simulink model "power_hvdc12pulse"  (Simulink 6.0)
settings: Solver=FixedStepDiscrete  SolverMode=SingleTasking  StartTime=0.0  StopTime=2  FixedStep=Ts  RelTol=1e-3  AbsTol=1e-2
InitFcn:
  | Ts=50e-6;
undefined symbols (not defined in the file or in its folder): CLARK, Current, D1, Delta, DiscIntNeverNeededParam, Gamma, Inverter, lag, lib_mesures, Voltage, Yg
libraries: powerlib x39, powerlib_extras x30, simulink x3
(part 1 of 3)
Description:
  | The 'Model  initialization function' defined in the
  | 
  | Model Properties automatically sets the sample time
  | 
  | Ts to 50e-6 s
settings Model: Creator=Gilbert Sybille, IREQ  LastModifiedBy=batserve  ExtModeTrigMode=oneshot  ExtModeArmWhenConnect=off  ExtModeAutoUpdateStatusClock=off
settings DataIOCC: LimitDataPoints=off  SaveTime=off  SignalLoggingName=sigsOut
settings OptimizationCC: BlockReduction=off  BooleanDataType=off
settings DebuggingCC: CheckExecutionContextPreStartOutputMsg=on  CheckExecutionContextRuntimeOutputMsg=on  SolverPrmCheckMsg=none  UnconnectedInputMsg=none  UnconnectedOutputMsg=none
settings HardwareCC: TargetUnknown=on

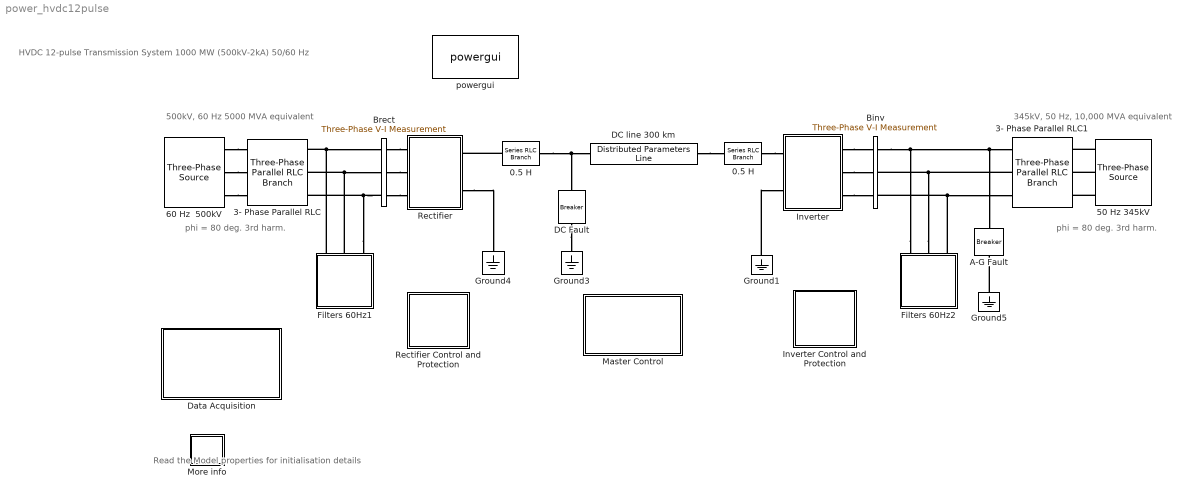
== system power_hvdc12pulse ==
  note: phi = 80 deg. 3rd harm.
  note: HVDC 12-pulse Transmission System
      | 1000 MW (500kV-2kA)   50/60 Hz
  note: 500kV, 60 Hz
      |  5000 MVA equivalent
  note: 345kV, 50 Hz,
      | 10,000 MVA equivalent
  note: phi = 80 deg. 3rd harm.
  note: Read the Model properties
      | for initialisation details
  " 50 Hz 345kV  " : powerlib/Electrical Sources/Three-Phase Source  Orientation=left  Voltage=345e3  PhaseAngle=0  Frequency=50  InternalConnection=Yg  SpecifyImpedance=off  Resistance=0  Inductance=28.0e-3  ShortCircuitLevel=0  BaseVoltage=0  XRratio=0
  " 60 Hz  500kV" : powerlib/Electrical Sources/Three-Phase Source  Voltage=500e3  PhaseAngle=0  Frequency=60  InternalConnection=Yg  SpecifyImpedance=off  Resistance=0  Inductance=98.03e-3  ShortCircuitLevel=0  BaseVoltage=0  XRratio=0
  0.5 H : powerlib/Elements/Series RLC Branch  PhysicalDomain=powersysdomain  SubClassName=unknown  LeftPortType=p1  RightPortType=p1  LConnTagsString=__new0  RConnTagsString=__new0  Resistance=1  Inductance=0.5  Capacitance=inf  Measurements=None
  "0.5 H " : powerlib/Elements/Series RLC Branch  Orientation=left  PhysicalDomain=powersysdomain  SubClassName=unknown  LeftPortType=p1  RightPortType=p1  LConnTagsString=__new0  RConnTagsString=__new0  Resistance=1  Inductance=0.5  Capacitance=inf  Measurements=None
  3- Phase Parallel RLC : powerlib/Elements/Three-Phase Parallel RLC Branch  PhysicalDomain=powersysdomain  SubClassName=unknown  LeftPortType=p1  RightPortType=p1  LConnTagsString=A|B|C  RConnTagsString=A|B|C  Resistance=26.07  Inductance=48.86e-3  Capacitance=0  Measurements=None
  3- Phase Parallel RLC1 : powerlib/Elements/Three-Phase Parallel RLC Branch  Orientation=left  PhysicalDomain=powersysdomain  SubClassName=unknown  LeftPortType=p1  RightPortType=p1  LConnTagsString=A|B|C  RConnTagsString=A|B|C  Resistance=6.205  Inductance=13.96e-3  Capacitance=0  Measurements=None
  A-G Fault : powerlib/Elements/Breaker  Orientation=down  BreakerResistance=0.01  InitialState=0  SnubberResistance=inf  SnubberCapacitance=inf  SwitchingTimes=[ 0.7 0.8]*100  External=off  Measurements=Branch current
      settings: AttributesFormatString=\n
  Binv : powerlib/Measurements/Three-Phase V-I Measurement  Orientation=left  VoltageMeasurement=phase-to-ground  SetLabelV=on  LabelV=Vabc_I  Vpu=on  Vbase=345e3  CurrentMeasurement=yes  SetLabelI=on  LabelI=Iabc_I  Ipu=on  Pbase=100e6  OutputType=Magnitude  PhasorSimulation=off  PSBequivalent=0
  Brect : powerlib/Measurements/Three-Phase V-I Measurement  VoltageMeasurement=phase-to-ground  SetLabelV=on  LabelV=Vabc_R  Vpu=on  Vbase=500e3  CurrentMeasurement=yes  SetLabelI=on  LabelI=Iabc_R  Ipu=on  Pbase=100e6  OutputType=Magnitude  PhasorSimulation=off  PSBequivalent=0
  DC Fault : powerlib/Elements/Breaker  Orientation=down  BreakerResistance=1  InitialState=0  SnubberResistance=inf  SnubberCapacitance=inf  SwitchingTimes=[0.7 0.75]*100  External=off  Measurements=Branch current
      settings: AttributesFormatString=\n
  DC line 300 km : powerlib/Elements/Distributed Parameters Line  Phases=1  Frequency=60  Resistance=0.015  Inductance=0.792e-3  Capacitance=14.4e-9  Length=300  x1=[0 -2.16105063708639e-012;0.000202625960824372 -2.78820694913162e-012;0.000405251921648744 -3.41415596345104e-012;0.000607877882473116 -4.03596541237589e-012;0.000810503843297489 -4.65066327836032e-012;0.00101312980412186 -5.25525247617399e-012]  x2=[0 -1.28636510443273e-012;0.000202625960824372 -1.90237836086429e-012;0.000405251921648744 -2.52160651295295e-012;0.000607877882473116 -3.14111601303326e-012;0.000810503843297489 -3.75791095814674e-012;0.00101312980412186 -4.36894806263535e-012]  x3=[0 -5.39692178751901e-015;0.000202625960824372 -7.25920757796091e-015;0.000405251921648744 -9.14272797774125e-015;0.000607877882473116 -1.10394956670709e-014;0.000810503843297489 -1.29411763980793e-014;0.00101312980412186 -1.48391265509203e-014]  x4=[0 4.1267112956018e-015;0.000202625960824372 8.19507726484828e-016;0.000405251921648744 -2.53679729362182e-015;0.000607877882473116 -5.92679713170551e-015;0.000810503843297489 -9.33469221052342e-015;0.00101312980412186 -1.27443660669749e-014]  x5=0.00101312980412186  Measurements=Phase-to-ground voltages
      settings: AttributesFormatString=\n
  Data Acquisition : Subsystem
      mask Display: disp('Open this block\nto visualize\nrecorded signals')
  Filters 60Hz1 : Subsystem  Orientation=down
      mask Display: disp('AC filters \n60 Hz\n600 Mvar')
  Filters 60Hz2 : Subsystem  Orientation=down
      mask Display: disp('AC filters \n50 Hz\n600 Mvar')
  Ground{1,3..5} (4 alike) : powerlib/Elements/Ground  Orientation=down  PhysicalDomain=powersysdomain  SubClassName=unknown  LeftPortType=p1  RightPortType=p1  LConnTagsString=a
  Inverter : Subsystem  Orientation=left
  Inverter Control and Protection : Subsystem  Orientation=left
  Master Control : Subsystem
      mask Display: disp('Master Control')
  More info : Subsystem
      mask Display: disp('?')
  Rectifier : Subsystem
  Rectifier Control and Protection : Subsystem
  powergui : powerlib/powergui  Priority=2  Frange=[0:2:500]  Ylog=off  Xlog=on  save=off  variable=ZData  ZoomFFT=on  StartTime=0.0  cycles=1  DisplayStyle=off  fundamental=60  FreqAxis=off  MaxFrequency=1000  frequencyindice=1  frequencyindicesteady=1  RmsSteady=1  display=off  Ts=Ts  methode=off  frequency=60  echomessages=on
  connections:
  DC Fault/RConn1 -- Ground3/LConn1
  " 60 Hz  500kV"/RConn1 -- 3- Phase Parallel RLC/LConn1
  " 60 Hz  500kV"/RConn2 -- 3- Phase Parallel RLC/LConn2
  " 60 Hz  500kV"/RConn3 -- 3- Phase Parallel RLC/LConn3
  Filters 60Hz1/LConn2 -- 3- Phase Parallel RLC/RConn2 -- Brect/LConn2
  Filters 60Hz1/LConn3 -- Brect/LConn3 -- 3- Phase Parallel RLC/RConn3
  " 50 Hz 345kV  "/RConn2 -- 3- Phase Parallel RLC1/LConn2
  " 50 Hz 345kV  "/RConn1 -- 3- Phase Parallel RLC1/LConn1
  " 50 Hz 345kV  "/RConn3 -- 3- Phase Parallel RLC1/LConn3
  Filters 60Hz2/LConn1 -- 3- Phase Parallel RLC1/RConn1 -- A-G Fault/LConn1 -- Binv/LConn1
  Filters 60Hz2/LConn2 -- 3- Phase Parallel RLC1/RConn2 -- Binv/LConn2
  Filters 60Hz2/LConn3 -- 3- Phase Parallel RLC1/RConn3 -- Binv/LConn3
  Filters 60Hz1/LConn1 -- 3- Phase Parallel RLC/RConn1 -- Brect/LConn1
  Rectifier/RConn2 -- Ground4/LConn1
  Ground1/LConn1 -- Inverter/RConn2
  Ground5/LConn1 -- A-G Fault/RConn1
  Inverter/LConn1 -- Binv/RConn1
  Inverter/LConn2 -- Binv/RConn2
  Inverter/LConn3 -- Binv/RConn3
  Brect/RConn1 -- Rectifier/LConn1
  Brect/RConn2 -- Rectifier/LConn2
  Brect/RConn3 -- Rectifier/LConn3
  0.5 H/LConn1 -- Rectifier/RConn1
  DC line 300 km/RConn1 -- "0.5 H "/RConn1
  "0.5 H "/LConn1 -- Inverter/RConn1
  0.5 H/RConn1 -- DC line 300 km/LConn1 -- DC Fault/LConn1

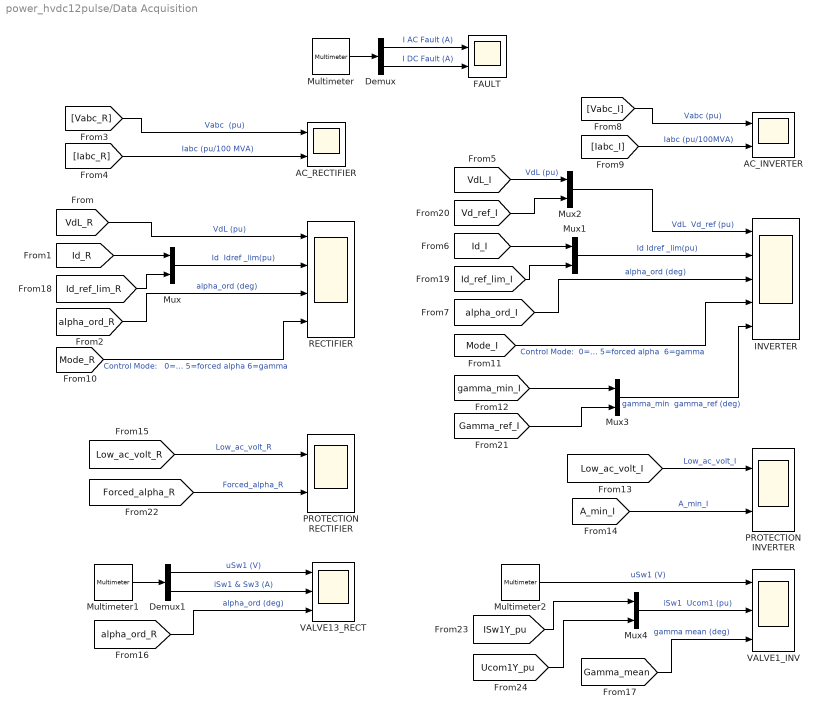
== system power_hvdc12pulse/Data Acquisition ==
  AC_INVERTER : Scope  NumInputPorts=2
      settings: YMin=-1.25~-50  YMax=1.5~20  SaveName=VI_abc_inv  Decimation=Ts  SampleInput=on  SampleTime=Ts
  AC_RECTIFIER : Scope  NumInputPorts=2
      settings: TimeRange=0.2008622476996453  YMin=-1~-25  YMax=1~30  DataFormat=Array  Decimation=Ts  SampleInput=on  SampleTime=Ts
  Demux : Demux  Outputs=2
  Demux1 : Demux  Outputs=[1 2]
  FAULT : Scope  NumInputPorts=2
      settings: YMin=-1~-1000  YMax=1~8000  Decimation=Ts  SampleInput=on  SampleTime=Ts
  INVERTER : Scope  NumInputPorts=5
      settings: TimeRange=2  YMin=-0.5~-0.5~50~0~0  YMax=1.5~1.5~200~6~200  SaveName=inv  Decimation=Ts  SampleInput=on  SampleTime=Ts
  Multimeter : powerlib/Measurements/Multimeter  Tag=PoWeRsYsTeMmEaSuReMeNt  PhasorSimulation=off  OutputType=Magnitude  sel=[23 24]  L=42  Gain=[1 1]  yselected={'Ib: A-G Fault','Ib: DC Fault'};  PSBOutputType=1  PSBequivalent=0  AxesSetting=[0,0.1,-100,100]  Display=0  SavedBlockNames={}
      settings: AttributesFormatString=\n
  Multimeter1 : powerlib/Measurements/Multimeter  Tag=PoWeRsYsTeMmEaSuReMeNt  PhasorSimulation=off  OutputType=Magnitude  sel=[11 37 39]  L=42  Gain=[1 1 1]  yselected={'Usw1: Rectifier/Rectifier/Bridge Y','Isw1: Rectifier/Rectifier/Bridge Y','Isw3: Rectifier/Rectifier/Bridge Y'};  PSBOutputType=1  PSBequivalent=0  AxesSetting=[0,0.1,-100,100]  Display=0  SavedBlockNames={}
      settings: AttributesFormatString=\n
  Multimeter2 : powerlib/Measurements/Multimeter  Tag=PoWeRsYsTeMmEaSuReMeNt  PhasorSimulation=off  OutputType=Magnitude  sel=1  L=42  Gain=1  yselected={'Usw1: Inverter/Inverter/Bridge Y'};  PSBOutputType=1  PSBequivalent=0  AxesSetting=[0,0.1,-100,100]  Display=0  SavedBlockNames={}
      settings: AttributesFormatString=\n
  Mux{,1..4} (5 alike) : Mux  Inputs=2
  PROTECTION INVERTER : Scope  NumInputPorts=2
      settings: YMin=-1~2.71051e-020  YMax=1~0.0007  SaveName=ScopeData2  DataFormat=Array  Decimation=Ts  SampleInput=on  SampleTime=Ts
  PROTECTION RECTIFIER : Scope  NumInputPorts=2
      settings: YMin=-1.25~-5  YMax=1.25~5  SaveName=ScopeData5  DataFormat=Array  Decimation=Ts  SampleInput=on  SampleTime=Ts
  RECTIFIER : Scope  NumInputPorts=4
      settings: YMin=-0.5~-0.1~0~0  YMax=1.25~1.1~175~5  SaveName=rect  Decimation=Ts  SampleInput=on  SampleTime=Ts
  VALVE13_RECT : Scope  NumInputPorts=3
      settings: YMin=-400000~-500~10  YMax=400000~2500~100  SaveName=ScopeData3  Decimation=Ts  SampleInput=on  SampleTime=Ts
  VALVE1_INV : Scope  NumInputPorts=3
      settings: YMin=-200000~-2~-1  YMax=350000~2~1  SaveName=ScopeData6  Decimation=Ts  SampleInput=on  SampleTime=Ts
  wires:
  [Mode_R] -> RECTIFIER/4  "Control Mode:   0=blocked  1=current 2=voltage 3=alpha min  4=alpha max 5=forced alpha 6=gamma"
  Demux/2 -> FAULT/2  "I DC Fault (A)"
  Demux/1 -> FAULT/1  "I AC Fault (A)"
  [alpha_ord_I] -> INVERTER/3  "alpha_ord (deg)"
  [Iabc_I] -> AC_INVERTER/2  "Iabc (pu/100MVA)"
  [Vabc_I] -> AC_INVERTER/1  "Vabc (pu)"
  [alpha_ord_R] -> RECTIFIER/3  "alpha_ord (deg)"
  [VdL_R] -> RECTIFIER/1  "VdL (pu)"
  [Iabc_R] -> AC_RECTIFIER/2  "Iabc (pu/100 MVA)"
  [Vabc_R] -> AC_RECTIFIER/1  "Vabc  (pu)"
  Multimeter/1 -> Demux/1
  [Low_ac_volt_I] -> PROTECTION INVERTER/1  "Low_ac_volt_I"
  [A_min_I] -> PROTECTION INVERTER/2  "A_min_I"
  [Low_ac_volt_R] -> PROTECTION RECTIFIER/1  "Low_ac_volt_R"
  Mux/1 -> RECTIFIER/2  "Id  Idref _lim(pu)"
  [Id_R] -> Mux/1
  [Id_ref_lim_R] -> Mux/2
  [Id_I] -> Mux1/1
  [Id_ref_lim_I] -> Mux1/2
  Mux1/1 -> INVERTER/2  "Id Idref _lim(pu)"
  [Mode_I] -> INVERTER/4  "Control Mode:  0=blocked  1=current  2=voltage  3=alpha min  4=alpha max  5=forced alpha  6=gamma"
  [VdL_I] -> Mux2/1  "VdL (pu)"
  Mux2/1 -> INVERTER/1  "VdL  Vd_ref (pu)"
  [Vd_ref_I] -> Mux2/2
  [gamma_min_I] -> Mux3/1
  Mux3/1 -> INVERTER/5  "gamma_min  gamma_ref (deg)"
  [Gamma_ref_I] -> Mux3/2
  [Forced_alpha_R] -> PROTECTION RECTIFIER/2  "Forced_alpha_R"
  Multimeter1/1 -> Demux1/1
  Demux1/1 -> VALVE13_RECT/1  "uSw1 (V)"
  Demux1/2 -> VALVE13_RECT/2  "iSw1 & Sw3 (A)"
  [alpha_ord_R] -> VALVE13_RECT/3  "alpha_ord (deg)"
  Multimeter2/1 -> VALVE1_INV/1  "uSw1 (V)"
  [Gamma_mean] -> VALVE1_INV/3  "gamma mean (deg)"
  Mux4/1 -> VALVE1_INV/2  "iSw1  Ucom1 (pu)"
  [ISw1Y_pu] -> Mux4/1
  [Ucom1Y_pu] -> Mux4/2

== system power_hvdc12pulse/Filters 60Hz1 ==
  note: Capacitor banks
  note: Tuned filters
  note: High-pass
      | damped filter
  note: 60 Hz filters 4*150 Mvars @ 500 kV
  11th 150 Mvar Q=100 : powerlib/Elements/Three-Phase Harmonic Filter  Orientation=down  PhysicalDomain=powersysdomain  SubClassName=unknown  LeftPortType=p1  RightPortType=p1  LConnTagsString=A|B|C  FilterType=Single-tuned  FilterConnection=Y (grounded)  ParNom=[500e3 60]  Qc=150e6  Fr=[11*60]  Frd=[11*60 13*60]  Q=100  Measurements=None
      settings: AttributesFormatString=\n
  "13th 150 Mvar Q=100 " : powerlib/Elements/Three-Phase Harmonic Filter  Orientation=down  PhysicalDomain=powersysdomain  SubClassName=unknown  LeftPortType=p1  RightPortType=p1  LConnTagsString=A|B|C  FilterType=Single-tuned  FilterConnection=Y (grounded)  ParNom=[500e3 60]  Qc=150e6  Fr=[13*60]  Frd=[11*60 13*60]  Q=100  Measurements=None
      settings: AttributesFormatString=\n
  150 Mvar : powerlib/Elements/Three-Phase Series RLC Load  Orientation=down  PhysicalDomain=powersysdomain  SubClassName=unknown  LeftPortType=p1  RightPortType=p1  LConnTagsString=A|B|C  Configuration=Y (grounded)  NominalVoltage=500e3  NominalFrequency=60  ActivePower=0  InductivePower=0  CapacitivePower=150e6  Measurements=None
  24th 150 Mvar Q=3 : powerlib/Elements/Three-Phase Harmonic Filter  Orientation=down  PhysicalDomain=powersysdomain  SubClassName=unknown  LeftPortType=p1  RightPortType=p1  LConnTagsString=A|B|C  FilterType=High-pass  FilterConnection=Y (grounded)  ParNom=[500e3 60]  Qc=150e6  Fr=[24*60]  Frd=[11*60 13*60]  Q=3  Measurements=None
      settings: AttributesFormatString=\n
  A : PMIOPort  Orientation=down  Port=1  Side=Left
  B : PMIOPort  Orientation=down  Port=2  Side=Left
  C : PMIOPort  Orientation=down  Port=3  Side=Left
  connections:
  150 Mvar/LConn3 -- 24th 150 Mvar Q=3/LConn3 -- "13th 150 Mvar Q=100 "/LConn3 -- 11th 150 Mvar Q=100/LConn3 -- C/RConn1
  150 Mvar/LConn2 -- 24th 150 Mvar Q=3/LConn2 -- "13th 150 Mvar Q=100 "/LConn2 -- 11th 150 Mvar Q=100/LConn2 -- B/RConn1
  150 Mvar/LConn1 -- 24th 150 Mvar Q=3/LConn1 -- "13th 150 Mvar Q=100 "/LConn1 -- 11th 150 Mvar Q=100/LConn1 -- A/RConn1

== system power_hvdc12pulse/Filters 60Hz2 ==
  note: 50 Hz filters 4*150 Mvars @ 345 kV
  note: Tuned filters
  note: Capacitor banks
  note: High-pass
      | damped filter
  11th 150 Mvar Q=100 : powerlib/Elements/Three-Phase Harmonic Filter  Orientation=down  PhysicalDomain=powersysdomain  SubClassName=unknown  LeftPortType=p1  RightPortType=p1  LConnTagsString=A|B|C  FilterType=Single-tuned  FilterConnection=Y (grounded)  ParNom=[345e3 50]  Qc=150e6  Fr=[11*50]  Frd=[11*60 13*60]  Q=100  Measurements=None
      settings: AttributesFormatString=\n
  "13th 150 Mvar Q=100 " : powerlib/Elements/Three-Phase Harmonic Filter  Orientation=down  PhysicalDomain=powersysdomain  SubClassName=unknown  LeftPortType=p1  RightPortType=p1  LConnTagsString=A|B|C  FilterType=Single-tuned  FilterConnection=Y (grounded)  ParNom=[345e3 50]  Qc=150e6  Fr=[13*50]  Frd=[11*60 13*60]  Q=100  Measurements=None
      settings: AttributesFormatString=\n
  150 Mvar : powerlib/Elements/Three-Phase Series RLC Load  Orientation=down  PhysicalDomain=powersysdomain  SubClassName=unknown  LeftPortType=p1  RightPortType=p1  LConnTagsString=A|B|C  Configuration=Y (grounded)  NominalVoltage=345e3  NominalFrequency=50  ActivePower=0  InductivePower=0  CapacitivePower=150e6  Measurements=None
  24th 150 Mvar Q=3 : powerlib/Elements/Three-Phase Harmonic Filter  Orientation=down  PhysicalDomain=powersysdomain  SubClassName=unknown  LeftPortType=p1  RightPortType=p1  LConnTagsString=A|B|C  FilterType=High-pass  FilterConnection=Y (grounded)  ParNom=[345e3 50]  Qc=150e6  Fr=[24*50]  Frd=[11*60 13*60]  Q=3  Measurements=None
      settings: AttributesFormatString=\n
  A : PMIOPort  Orientation=down  Port=1  Side=Left
  B : PMIOPort  Orientation=down  Port=2  Side=Left
  C : PMIOPort  Orientation=down  Port=3  Side=Left
  connections:
  150 Mvar/LConn1 -- 24th 150 Mvar Q=3/LConn1 -- "13th 150 Mvar Q=100 "/LConn1 -- 11th 150 Mvar Q=100/LConn1 -- A/RConn1
  150 Mvar/LConn2 -- 24th 150 Mvar Q=3/LConn2 -- "13th 150 Mvar Q=100 "/LConn2 -- 11th 150 Mvar Q=100/LConn2 -- B/RConn1
  150 Mvar/LConn3 -- 24th 150 Mvar Q=3/LConn3 -- "13th 150 Mvar Q=100 "/LConn3 -- 11th 150 Mvar Q=100/LConn3 -- C/RConn1

== system power_hvdc12pulse/Inverter ==
  1200 MVA : powerlib/Elements/Three-Phase Transformer (Three Windings)  Orientation=left  NominalPower=[ 1200e6 , 50 ]  Winding1Connection=Yg  Winding1="[ 345e3*0.96 0.0025  0 ]"  Winding2Connection=Y  Winding2="[ 200e3  0.0025 0.24]"  Winding3Connection=Delta (D1)  Winding3=[ 200e3 0.0025 0.24 ]  SetSaturation=off  Rm=500  Lm=500  Saturation="[0 0; 0.0024 1.2; 1.0  1.45]"  Hysteresis=off  DataFile='hysteresis'  SetInitialFlux=off  InitialFluxes=[-1.10749033878531 0.564800371868647 0.542689966916658]  Measurements=None  TransfoNumber=0
      settings: AttributesFormatString=\n
  A->pu : Gain  Orientation=left  Gain=1/2000  SaturateOnIntegerOverflow=on
  Id : powerlib/Measurements/Current Measurement  Tag=PoWeRsYsTeMmEaSuReMeNt  PhasorSimulation=off  OutputType=Magnitude  PSBequivalent=0
  Inverter : Subsystem  Orientation=left
      mask Display: plot(0,0,100,100,[30 70 50 30 ], [60 60 40 60], [50 50], [25 40], [50 50], [ 60 75], [30 70], [40 40], [50 60 70], [40 30 30]);
  A : PMIOPort  Orientation=left  Port=1  Side=Left
  B : PMIOPort  Orientation=left  Port=2  Side=Left
  C : PMIOPort  Orientation=left  Port=3  Side=Left
  + : PMIOPort  Port=4  Side=Right
  - : PMIOPort  Port=5  Side=Right
  tag scope: Id_I=global
  wires:
  [PulsesY_I] -> Inverter/1(Py)
  [PulsesD_I] -> Inverter/2(Pd)
  Id/1 -> A->pu/1
  A->pu/1 -> [Id_I]
  connections:
  C/RConn1 -- 1200 MVA/LConn3
  A/RConn1 -- 1200 MVA/LConn1
  -/RConn1 -- Inverter/RConn2
  Inverter/LConn6 -- 1200 MVA/RConn6
  1200 MVA/RConn5 -- Inverter/LConn5
  Inverter/LConn4 -- 1200 MVA/RConn4
  1200 MVA/RConn3 -- Inverter/LConn3
  Inverter/LConn2 -- 1200 MVA/RConn2
  1200 MVA/RConn1 -- Inverter/LConn1
  1200 MVA/LConn2 -- B/RConn1
  +/RConn1 -- Id/LConn1
  Id/RConn1 -- Inverter/RConn1

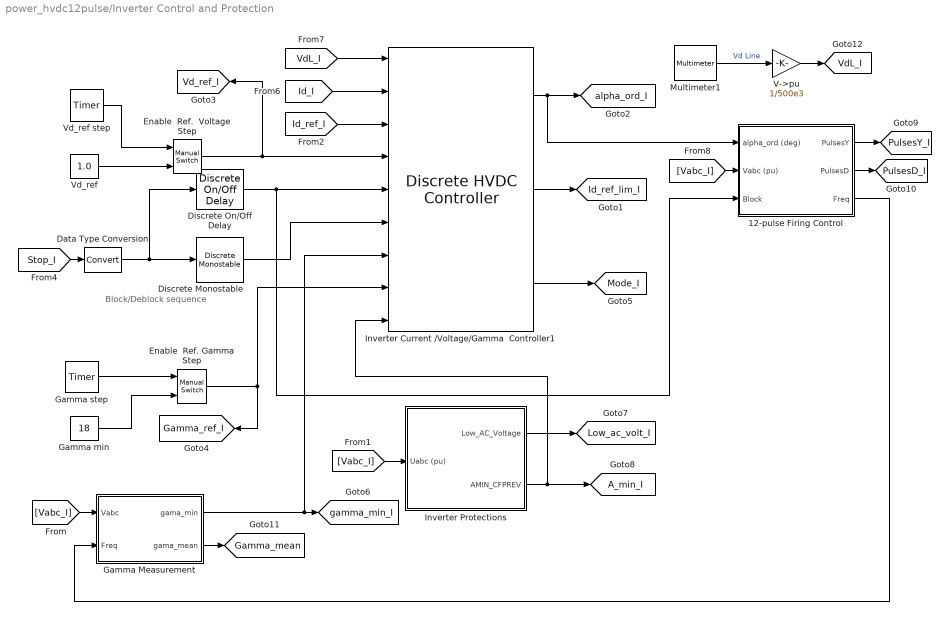
== system power_hvdc12pulse/Inverter Control and Protection ==
  note: Block/Deblock sequence
  12-pulse Firing Control : Subsystem  mask(HVDC Discrete 12-pulse Firing Control){Pw=101.5, PLL_PF=[0,  50], PLL_G=[60, 1400], dt=Ts}
      mask prompts: Pw "{Pulse Generator}: Pulse Width (deg)"; PLL_PF "{PLL}: Initial [Phase (deg) Frequency (Hz)]"; PLL_G "{PLL}: Regulator gains [Kp (rad)  Ki (rad/s)]"; dt "Sample Time (s):"
      mask help:
      | This block contains a PLL and a 12-pulse generator to provide the firing pulses to the HVDC converter.
      | The firing control is of the equidistant type. It is based on a Phase Locked Loop (PLL) synchronized on positive-sequence of the fundamental voltage.
      mask init:
      | PLL_ph = PLL_PF(1); PLL_f0 = PLL_PF(2);
      | PLL_Kp = PLL_G(1); PLL_Ki = PLL_G(2);
      mask Help:
      | INPUTS:
      | alpha :  Desired firing angle of thyristors (deg).
      | Vabc  : 3 phase-to-ground voltages (pu)  on the primary winding of the YgYD converter transformer
      | Block  : Logical signal  (0-1). The pulses are not generated when the value is 1.
      | 
      | 
      | 
      | OUTPUTS:
      |  PulsesY :  6 pulses to be sent to the half converter connected to the Wye winding.
      |  PulsesD :  6 pulses to be sent to the half converter connected to the Delta winding.
  Data Type Conversion : DataTypeConversion  OutDataTypeMode=boolean  SaturateOnIntegerOverflow=on  RndMeth=Zero
  Discrete Monostable : powerlib_extras/Discrete  Control Blocks/Discrete Monostable  EdgeDetect=Rising  t_mono=0.15  ic=1  Ts=Ts
  Discrete On/Off Delay : powerlib_extras/Discrete  Control Blocks/Discrete On//Off Delay  type_delay=On delay  delay=0.1  ic=1  Ts=Ts
  Enable  Ref.  Voltage Step : simulink/Signal Routing/Manual Switch  sw=1  action=0
  Enable  Ref. Gamma Step : simulink/Signal Routing/Manual Switch  sw=0  action=0
  Gamma Measurement : Subsystem
  Gamma min : Constant  Value=18
  Gamma step : powerlib_extras/Control  Blocks/Timer  t="[ 0  0.7  0.9  ]"  e="[ 18   23   18  ]"
  Inverter Current /Voltage/Gamma  Controller1 : powerlib_extras/Discrete  Control Blocks/Discrete HVDC Controller  Mode=Inverter (Current + Voltage + Gamma)  XPILim=[166, 92]  XLin=[160, 120]  XKPI_I=[45, 4500, 90]  Id_marg=0.1  XKPI_V="[35, 2250,  90]"  Vd_marg=0.05  XKPI_G="[1, 20,  90 ]"  G_marg=1  T_I=0.3e-3  XT_V="[15,  0.707]"  Xvdcol=[0.6, 0.18, 0.30, 0.1, 0.080]  alpha_const=off  Xalpha_fix=[92, inf, -1000]  dt=Ts
  Inverter Protections : Subsystem  TreatAsAtomicUnit=on
      mask Type: Protection LACVD a Radisson (cyc = 1 ms)
  Multimeter1 : powerlib/Measurements/Multimeter  Tag=PoWeRsYsTeMmEaSuReMeNt  PhasorSimulation=off  OutputType=Magnitude  sel=22  L=42  Gain=1  yselected={'Ur_ph1_gnd: DC line 300 km'};  PSBOutputType=1  PSBequivalent=0  AxesSetting=[0,0.1,-100,100]  Display=0  SavedBlockNames=-11
      settings: AttributesFormatString=\n
  V->pu : Gain  Gain=1/500e3  SaturateOnIntegerOverflow=on
  Vd_ref : Constant  Value=1.0
  Vd_ref step : powerlib_extras/Control  Blocks/Timer  t="[ 0  1  1.1  ]"  e="[ 1   0.9   1  ]"
  tag scope: A_min_I=global, Gamma_mean=global, Gamma_ref_I=global, Id_ref_lim_I=global, Low_ac_volt_I=global, Mode_I=global, PulsesD_I=global, PulsesY_I=global, VdL_I=global, Vd_ref_I=global, alpha_ord_I=global, gamma_min_I=global
  wires:
  Data Type Conversion/1 -> Discrete On/Off Delay/1, Discrete Monostable/1
  [Stop_I] -> Data Type Conversion/1
  [Vabc_I] -> Inverter Protections/1(Uabc (pu))
  Inverter Protections/2(AMIN_CFPREV) -> [A_min_I], Inverter Current /Voltage/Gamma  Controller1/9
  Inverter Protections/1(Low_AC_Voltage) -> [Low_ac_volt_I]
  V->pu/1 -> [VdL_I]
  Multimeter1/1 -> V->pu/1  "Vd Line"
  Enable  Ref. Gamma Step/1 -> [Gamma_ref_I], Inverter Current /Voltage/Gamma  Controller1/8
  Gamma step/1 -> Enable  Ref. Gamma Step/1
  Gamma min/1 -> Enable  Ref. Gamma Step/2
  Gamma Measurement/1(gama_min) -> [gamma_min_I], Inverter Current /Voltage/Gamma  Controller1/7
  [Vabc_I] -> Gamma Measurement/1(Vabc)
  Gamma Measurement/2(gama_mean) -> [Gamma_mean]
  12-pulse Firing Control/1(PulsesY) -> [PulsesY_I]
  12-pulse Firing Control/2(PulsesD) -> [PulsesD_I]
  Inverter Current /Voltage/Gamma  Controller1/1 -> [alpha_ord_I], 12-pulse Firing Control/1(alpha_ord (deg))
  Inverter Current /Voltage/Gamma  Controller1/2 -> [Id_ref_lim_I]
  Inverter Current /Voltage/Gamma  Controller1/3 -> [Mode_I]
  [Vabc_I] -> 12-pulse Firing Control/2(Vabc (pu))
  [VdL_I] -> Inverter Current /Voltage/Gamma  Controller1/1
  [Id_I] -> Inverter Current /Voltage/Gamma  Controller1/2
  [Id_ref_I] -> Inverter Current /Voltage/Gamma  Controller1/3
  Discrete On/Off Delay/1 -> 12-pulse Firing Control/3(Block), Inverter Current /Voltage/Gamma  Controller1/5
  Enable  Ref.  Voltage Step/1 -> Inverter Current /Voltage/Gamma  Controller1/4, [Vd_ref_I]
  Vd_ref/1 -> Enable  Ref.  Voltage Step/2
  Vd_ref step/1 -> Enable  Ref.  Voltage Step/1
  Discrete Monostable/1 -> Inverter Current /Voltage/Gamma  Controller1/6
  12-pulse Firing Control/3(Freq) -> Gamma Measurement/2(Freq)

== system power_hvdc12pulse/Master Control ==
  note: Master Control
  note: Balanced reference currents
  Constant : Constant  Value=0
  Enable  Ref. Current Step : simulink/Signal Routing/Manual Switch  sw=1  action=0
  Id_ref step : powerlib_extras/Control  Blocks/Timer  t="[ 0  0.7  0.8  ]"  e="[ 0   -0.2   0  ]"
  Informations : Subsystem
      mask Display: disp('?')
  Start/Stop : Subsystem  mask(Start/Stop  & Ramping  ){Min_ref=0.1, X_start=[0.3333, 0.02], X_up=[5.0, 0.4, 1.0], X_down=[-5.0,  1.4], T_stop=1.6}
      mask prompts: Min_ref "Minimum Steady-State Current Reference (pu):"; X_start "{Start Ramp}: [Rate (pu/s), Time (s)]"; X_up "{Up Ramp}: [Rate (pu/s), Time (s), Final Value (pu)]"; X_down "{Down Ramp}: [Rate (-pu/s), Time (s)]"; T_stop "Stop Time (s):"
      mask help:
      | At start-up, both converters are deblocked and ramped up to the minimum current (Minimum Steady-State Current Reference) with an adjustable rate (Start Ramp Rate) and application time (Start Ramp Time).
      |
      | After the system stabilisation the current is ramped up to its final value (Up Ramp Final Value) with an adjustable rate (Up Ramp Rate) and execution time (Up Ramp Time).
      |
      | Before stopping the converters (at Stop Time) the current is ramped down to the minimum current  with an adjustable rate (Down Ramp Rate) and execution time  (Down Ramp Time).
      |
      | At Stop Time the reference is ramped down to zero with the same rate used for the Start Ramp.
      mask init:
      | T_up = X_up(2); F_up = X_up(3); up_slope = X_up(1);
      | T_up_final =  T_up + (F_up - Min_ref)/up_slope;
      | 
      | T_down = X_down(2); F_down = Min_ref; down_slope = X_down(1);
      | T_down_final =   T_down + (F_down-F_up)/down_slope;
      | 
      | SS_ramp = X_start(1); T_start = X_start(2);
      | 
      | T_ramp  = [0, T_up, T_up_final,  T_down,  T_down_final, 9999]';
      | U_ramp = [0, 0, F_up-Min_ref,  F_up-Min_ref,  F_down- Min_ref,  F_down - Min_ref]';
      mask Display: disp('Start/Stop\n & Ramping')
  Sum : Sum  SaturateOnIntegerOverflow=on
  tag scope: Id_ref_I=global, Id_ref_R=global, Stop_I=global, Stop_R=global
  wires:
  Id_ref step/1 -> Enable  Ref. Current Step/1
  Constant/1 -> Enable  Ref. Current Step/2
  Enable  Ref. Current Step/1 -> Sum/2
  Sum/1 -> [Id_ref_R], [Id_ref_I]
  Start/Stop/2("Stop ") -> [Stop_I], [Stop_R]
  Start/Stop/1(Id_ref_ramp) -> Sum/1

== system power_hvdc12pulse/More info ==
  note: In the DC Fault block, change the multiplication factor of 1 in the Switching times to 100, so that the DC fault is now eliminated. In the A-G Fault block, change to 1 the 100 multiplication factor in the
      | Switching times so that a 6 cycles  line-to-ground fault is now applied at t = 0.7 s. The Low AC voltage detection (LACVD) subsystem in the rectifier and inverter protections and the Commutation
      | Failure Prevention Control (CFPREV) in the inverter protection are activated by default. Restart the simulation.
      |
      | Notice the 120 Hz oscillations in the DC voltage and currents during the fault. When the fault is cleared at t = 0.8 s,  the VDCOL operates and reduces the reference current to 0.3 pu. The system
      | recovers in approximately 0.35 s after fault clearing.  The  LACVD detects the fault and locks the DC Fault  protection  that should not detect a DC fault even if the DC line voltage dips.  Look at the
      | CFPREV output (A_min_I) which decreases the maximum delay angle limit in order to increase the commutation margin during and after the fault. Now deactivate the CFPREV protection by
      | deselecting  the "ON State" in the CFPREV dilaog box. Restart the simulation and observe the difference in  recovery time of the DC transmission. Note that a  commutation failure now occurs during
      | the recovery.  A commutation failure is the result of a failure of the incoming valve to take over the direct current before the commutation voltage reverses its polarity.  The symptoms are  a zero DC
      | voltage accros the affected bridge  causing an increase of the DC current at a rate determined mainly by the DC circuit inductance.
  note: AC line-to-ground fault at the inverter
  note: Deactivate the steps applied on the current reference and on the voltage reference in the Master Control and in the inverter control respectively by setting the switches in lower position. In the DC
      | Fault block, change to 1 the 100 multiplication factor in the Switching times so that a fault is now applied at t = 0.7 s. Reduce the Simulation stop time from 2 to 1.4 s. The DC Fault protection (DCPROT)
      | in the rectifier is activated by default. Open the FAULT scope to observe the DC fault current. Restart the simulation.
      |
      | At fault application the DC current quickly increases to 2.3 pu and the DC voltage falls to zero at the rectifier. This DC voltages drop is seen by the Voltage Dependant Currrent Order Limiter (VDCOL)
      | which reduces the reference current to 0.3 pu at the rectifier. A DC current still continues to circulate in the fault. Then, at t = 0.77 s, the rectifier alpha firing angle is forced to 166 degrees by the DC
      | protection because  a DC voltage drop is detected (VdL< 0.5 pu for more than 70 ms). The rectifier now operates in inverter mode. The DC line voltage becomes negative and the energy stored in the
      | line is returned to the AC network, causing rapid extinction of the fault current at its next zero-crossing. Then, alpha is released at t = 0.87 s and the normal DC voltage and current recover in
      | approximately 0.4 s.
  note: DC line fault at the rectifier
  note: Start-up and Stop
  note: DEMONSTRATION
  note: A 1000 MW (500 kV, 2kA) DC linterconnexion is used to transmit power from a 500 kV, 5000 MVA, 60 Hz network.
      | to a  345 kV, 10 000 MVA, 50 Hz network.
      |
      | The rectifier and the inverter are 12-pulse converters using two 6-pulse thyristor bridges connected in series. The rectifier and the inverter are interconnected through a 300 km distributed
      | parameter line and two 0.5 H smoothing reactors. The transformer tap changers are not simulated and  fixed taps are assumed. Open the two transformer blocks in the Rectifier and Inverter
      | subsystems to see the factors applied on the primary voltage: 0.90 on rectifier side and 0.96 on inverter side. Reactive power required by the converters is provided by a set of capacitor banks
      | plus 11th, 13th and  high pass filters for a total of  600 Mvar on each side. Two circuit breakers are used to apply faults on the inverter AC side and rectifier DC side.
      |
      | The rectifier and inverter control systems use the  Discrete 12-pulse HVDC Control block of the Extras/Discrete Control Blocks library. DC Protection functions are implemented in each converter.
      | At the rectifier the DC fault protection will detect and force the delay angle into the inverter region so to extinguish the fault current. At the inverter the commutation failure prevention control will
      | detect AC faults and reduce the maximum delay angle limit in order to decrease the risk of commutation failure. The Low AC voltage detection blocks will lock the DC fault protection when a drop in
      | the AC voltage is detected. The Master Control block initiates the starting and stopping of the converters as well as the ramping up and down of the current references. The power system and the
      | control system are both  discretized for a sample time Ts=50 us. Notice that the "Model initialization" function of the model  automatically sets Ts = 50e-6 in your Matlab workspace. A description of
      | the control systems is provided in the HVDC Transmission System Case Study of the User's Manual.
  note: Steady-state and transient performance of a 12-pulse,
      | 1000 MW (500 kV-2kA) 50/60 Hz HVDC transmission system
  note: CIRCUIT DESCRIPTION
  note: The system is programmed to start and  reach a steady state. Then steps are applied on the reference current of the rectifier and  on the inverter reference voltage in order to observe the dynamic
      | response  of the regulators. Finally, a stop sequence is initiated to bring the DC power down before blocking the converters. Start the simulation. Open the RECTIFIER and INVERTER scopes (in the
      | Data Acquisition subsystem) and observe the DC line voltage  on trace 1 (1pu = 500 kV) and the DC line current  (reference and mesured values)  on trace 2 (1pu = 2kA).
  note: Verify in the Master Control that the "Enable Ref. Current Step"  switch is in the upper position. This switch is used to apply a step on the reference voltage. Also verify that the  reference voltage
      | step is enabled in the Inverter Control. At t=0.7 s, a -0.2 pu step is first applied on the reference current (decrease from 1 pu  to 0.8 pu ) and at t=0.8 s,  the reference current is reset to its 1 pu
      | original value.The current stabilizes in  approximately 0.1 seconds. Steps are also  applied on the reference voltage of the inverter (-0.1 pu / +0.1 pu at t=1.0 s / 1.1s. )
  note: Step response of curent and voltage regulators
  note: Silvano Casoria (Hydro-Quebec)
  note: In the Master Control, the converters are deblocked and started by ramping the rectifier and inverter reference current. At t = 0.02 s (i.e. when the converters at deblocked), the reference current
      | is ramped to reach the minimum value of 0.1 pu in 0.3 s (0.33 pu/s). At the end of this first ramp (t = 0.32 s) the DC line is charged at its nominal voltage and DC voltage reaches steady-state. At
      | t= 0.4 s,  the reference current is ramped from 0.1 pu to 1 pu (2kA) in 0.18 s (5 pu/s). At the end of this starting sequence (t=0.58 s) , the DC current reaches steady state. The RECTIFIER then
      | controls the current and the INVERTER controls the voltage. In steady-state, the alpha firing angles (trace 3) are 16.5 degrees and 143 degrees respectively on the RECTIFIER and INVERTER sides.
      | The exctinction angle gamma (minimum value) is measured at the INVERTER  and shown in trace 4. In steady-state, the minimum value is between 22 and 24 degrees. The control mode of operation
      | (an  integer between 0 to 6) is shown in trace 4 (0= blocked; 1=Current control; 2=Voltage control; 3=Alpha minimum limitation;  4=Alpha maximum limitation; 5=Forced or constant alpha;
      | 6=Gamma control). At t = 1.4 s the Stop sequence is initiated by ramping down the current to 0.1 pu. At t = 1.6 s a Forced-alpha at the Rectifier extinguishes the current and at the Inverter the
      | Forced-alpha brings down the DC voltage. At t = 1.7 s the pulses are blocked in both converters.

== system power_hvdc12pulse/Rectifier ==
  1200 MVA : powerlib/Elements/Three-Phase Transformer (Three Windings)  NominalPower=[ 1200e6 , 60 ]  Winding1Connection=Yg  Winding1="[ 500e3*0.9 0.0025  0 ]"  Winding2Connection=Y  Winding2=[ 200e3 0.0025 0.24]  Winding3Connection=Delta (D1)  Winding3=[ 200e3 0.0025 0.24 ]  SetSaturation=off  Rm=500  Lm=500  Saturation="[0 0; 0.0024 1.2; 1.0  1.45]"  Hysteresis=off  DataFile='hysteresis'  SetInitialFlux=off  InitialFluxes=[-1.26114097729929 0.657669801639854 0.603471175659435]  Measurements=None  TransfoNumber=0
      settings: AttributesFormatString=\n
  A->pu : Gain  Gain=1/2000  SaturateOnIntegerOverflow=on
  Rectifier : Subsystem
      mask Display: plot(0,0,100,100,[30 70 50 30 ], [40 40 60 40], [50 50], [25 40], [50 50], [ 60 75], [30 70], [60 60], [50 40 30], [60 70 70]);
  idR : powerlib/Measurements/Current Measurement  Tag=PoWeRsYsTeMmEaSuReMeNt  PhasorSimulation=off  OutputType=Magnitude  PSBequivalent=0
  A : PMIOPort  Port=1  Side=Left
  B : PMIOPort  Port=2  Side=Left
  C : PMIOPort  Port=3  Side=Left
  "+ " : PMIOPort  Orientation=left  Port=4  Side=Right
  - : PMIOPort  Orientation=left  Port=5  Side=Right
  tag scope: Id_R=global
  wires:
  idR/1 -> A->pu/1
  A->pu/1 -> [Id_R]
  [PulsesY_R] -> Rectifier/1(Py)
  [PulsesD_R] -> Rectifier/2(Pd)
  connections:
  idR/RConn1 -- "+ "/RConn1
  Rectifier/RConn2 -- -/RConn1
  Rectifier/RConn1 -- idR/LConn1
  Rectifier/LConn6 -- 1200 MVA/RConn6
  1200 MVA/RConn5 -- Rectifier/LConn5
  Rectifier/LConn4 -- 1200 MVA/RConn4
  1200 MVA/RConn3 -- Rectifier/LConn3
  Rectifier/LConn2 -- 1200 MVA/RConn2
  1200 MVA/RConn1 -- Rectifier/LConn1
  A/RConn1 -- 1200 MVA/LConn1
  B/RConn1 -- 1200 MVA/LConn2
  C/RConn1 -- 1200 MVA/LConn3

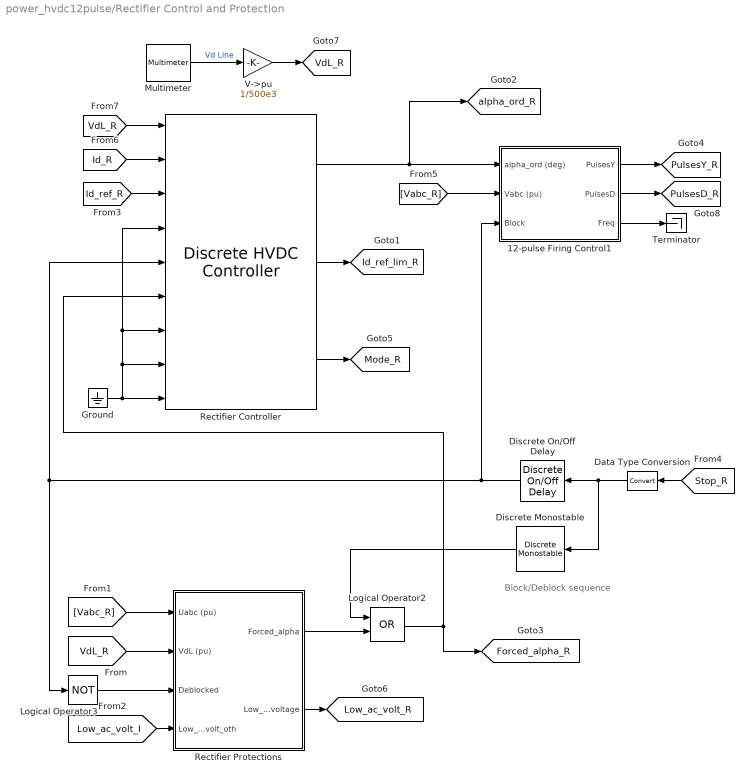
== system power_hvdc12pulse/Rectifier Control and Protection ==
  note: Block/Deblock sequence
  12-pulse Firing Control1 : Subsystem  mask(HVDC Discrete 12-pulse Firing Control){Pw=101.5, PLL_PF=[0,  50], PLL_G=[60, 1400], dt=Ts}
      mask prompts: Pw "{Pulse Generator}: Pulse Width (deg)"; PLL_PF "{PLL}: Initial [Phase (deg) Frequency (Hz)]"; PLL_G "{PLL}: Regulator gains [Kp (rad)  Ki (rad/s)]"; dt "Sample Time (s):"
      mask help:
      | This block contains a PLL and a 12-pulse generator to provide the firing pulses to the HVDC converter.
      | The firing control is of the equidistant type. It is based on a Phase Locked Loop (PLL) synchronized on positive-sequence of the fundamental voltage.
      mask init:
      | PLL_ph = PLL_PF(1); PLL_f0 = PLL_PF(2);
      | PLL_Kp = PLL_G(1); PLL_Ki = PLL_G(2);
      mask Help:
      | INPUTS:
      | alpha :  Desired firing angle of thyristors (deg).
      | Vabc  : 3 phase-to-ground voltages (pu)  on the primary winding of the YgYD converter transformer
      | Block  : Logical signal  (0-1). The pulses are not generated when the value is 1.
      | 
      | 
      | 
      | OUTPUTS:
      |  PulsesY :  6 pulses to be sent to the half converter connected to the Wye winding.
      |  PulsesD :  6 pulses to be sent to the half converter connected to the Delta winding.
  Data Type Conversion : DataTypeConversion  Orientation=left  OutDataTypeMode=boolean  SaturateOnIntegerOverflow=on  RndMeth=Zero
  Discrete Monostable : powerlib_extras/Discrete  Control Blocks/Discrete Monostable  Orientation=left  EdgeDetect=Rising  t_mono=0.15  ic=1  Ts=Ts
  Discrete On/Off Delay : powerlib_extras/Discrete  Control Blocks/Discrete On//Off Delay  Orientation=left  type_delay=On delay  delay=0.1  ic=1  Ts=Ts
  Ground : Ground
  Logical Operator2 : Logic  Operator=OR  AllPortsSameDT=off
  Logical Operator3 : Logic  Operator=NOT
  Multimeter : powerlib/Measurements/Multimeter  Tag=PoWeRsYsTeMmEaSuReMeNt  PhasorSimulation=off  OutputType=Magnitude  sel=21  L=42  Gain=1  yselected={'Us_ph1_gnd: DC line 300 km'};  PSBOutputType=1  PSBequivalent=0  AxesSetting=[0,0.1,-100,100]  Display=0  SavedBlockNames=-11
      settings: AttributesFormatString=\n
  Rectifier Controller : powerlib_extras/Discrete  Control Blocks/Discrete HVDC Controller  Mode=Rectifier (Current)  XPILim=[166, 5]  XLin=[160, 120]  XKPI_I=[45, 4500, 90]  Id_marg=0.1  XKPI_V="[35, 2250,  90]"  Vd_marg=0.05  XKPI_G="[1, 20,  90 ]"  G_marg=1  T_I=0.3e-3  XT_V="[15,  0.707]"  Xvdcol=[0.6, 0.18, 0.30, 0.1, 0.080]  alpha_const=off  Xalpha_fix=[166, inf, -inf]  dt=Ts
  Rectifier Protections : Subsystem  TreatAsAtomicUnit=on
      mask Type: Protection LACVD a Radisson (cyc = 1 ms)
  Terminator : Terminator
  V->pu : Gain  Gain=1/500e3  SaturateOnIntegerOverflow=on
  tag scope: Forced_alpha_R=global, Id_ref_lim_R=global, Low_ac_volt_R=global, Mode_R=global, PulsesD_R=global, PulsesY_R=global, VdL_R=global, alpha_ord_R=global
  wires:
  [Low_ac_volt_I] -> Rectifier Protections/4(Low_ac_volt_oth)
  Rectifier Protections/2(Low_ac_voltage) -> [Low_ac_volt_R]
  Discrete Monostable/1 -> Logical Operator2/1
  Discrete On/Off Delay/1 -> Logical Operator3/1, Rectifier Controller/5, 12-pulse Firing Control1/3(Block)
  Rectifier Protections/1(Forced_alpha) -> Logical Operator2/2
  Data Type Conversion/1 -> Discrete On/Off Delay/1, Discrete Monostable/1
  [Vabc_R] -> Rectifier Protections/1(Uabc (pu))
  [VdL_R] -> Rectifier Protections/2(VdL (pu))
  Logical Operator3/1 -> Rectifier Protections/3(Deblocked)
  [Stop_R] -> Data Type Conversion/1
  Ground/1 -> Rectifier Controller/4, Rectifier Controller/7, Rectifier Controller/8, Rectifier Controller/9
  [VdL_R] -> Rectifier Controller/1
  [Id_R] -> Rectifier Controller/2
  Rectifier Controller/1 -> [alpha_ord_R], 12-pulse Firing Control1/1(alpha_ord (deg))
  Rectifier Controller/2 -> [Id_ref_lim_R]
  Rectifier Controller/3 -> [Mode_R]
  Logical Operator2/1 -> [Forced_alpha_R], Rectifier Controller/6
  Multimeter/1 -> V->pu/1  "Vd Line"
  V->pu/1 -> [VdL_R]
  [Id_ref_R] -> Rectifier Controller/3
  12-pulse Firing Control1/1(PulsesY) -> [PulsesY_R]
  [Vabc_R] -> 12-pulse Firing Control1/2(Vabc (pu))
  12-pulse Firing Control1/2(PulsesD) -> [PulsesD_R]
  12-pulse Firing Control1/3(Freq) -> Terminator/1

== system power_hvdc12pulse/Inverter/Inverter ==
  Py : Inport  Port=1  LatchInput=off
  Pd : Inport  Port=2  LatchInput=off
  Bridge D : powerlib/Power Electronics/Universal Bridge  Arms=3  SnubberResistance=2000  SnubberCapacitance=0.1e-6  Device=Thyristors  Ron=1e-3  Lon=0  ForwardVoltages="[  0.8  0.8  ]"  ForwardVoltage=0  GTOparameters=[ 10e-6 , 20e-6 ]  IGBTparameters=[ 1e-6 , 2e-6 ]  Measurements=Device currents
  Bridge Y : powerlib/Power Electronics/Universal Bridge  Arms=3  SnubberResistance=2000  SnubberCapacitance=0.1e-6  Device=Thyristors  Ron=1e-3  Lon=0  ForwardVoltages="[  0.8  0.8  ]"  ForwardVoltage=0  GTOparameters=[ 10e-6 , 20e-6 ]  IGBTparameters=[ 1e-6 , 2e-6 ]  Measurements=All voltages and currents
  Ay : PMIOPort  Port=1  Side=Left
  By : PMIOPort  Port=2  Side=Left
  Cy : PMIOPort  Port=3  Side=Left
  Ad : PMIOPort  Port=4  Side=Left
  Bd : PMIOPort  Port=5  Side=Left
  Cd : PMIOPort  Port=6  Side=Left
  pos : PMIOPort  Orientation=left  Port=7  Side=Right
  neg : PMIOPort  Orientation=left  Port=8  Side=Right
  wires:
  Py/1 -> Bridge Y/1
  Pd/1 -> Bridge D/1
  connections:
  Bridge D/RConn1 -- neg/RConn1
  Bridge Y/RConn2 -- pos/RConn1
  Bridge D/RConn2 -- Bridge Y/RConn1
  Ay/RConn1 -- Bridge Y/LConn1
  By/RConn1 -- Bridge Y/LConn2
  Cy/RConn1 -- Bridge Y/LConn3
  Ad/RConn1 -- Bridge D/LConn1
  Bd/RConn1 -- Bridge D/LConn2
  Cd/RConn1 -- Bridge D/LConn3

== system power_hvdc12pulse/Inverter Control and Protection/12-pulse Firing Control ==
  alpha_ord (deg) : Inport  Port=1  LatchInput=off
  Vabc (pu) : Inport  Port=2  LatchInput=off
  Block : Inport  Port=3  LatchInput=off
  Discrete Synchronized 12-Pulse Generator : Subsystem  AncestorBlock=|  mask(Discrete synchronized 12-pulse generator){pwidth=Pw, Double_Pulse=off, Ts=dt}
      | powerlib_extras/Discrete 
      | Control Blocks/Discrete Synchronized
      | 12-Pulse Generator
      mask prompts: pwidth "Pulse width (degrees) :"; Double_Pulse "Double pulsing"; Ts "Sample time:"
      mask help:
      | Use his block  to fire the 12 thyristors of a 12-pulse converter.
      | Outputs 1 and 2 are two vectors of 6 pulses (0-1) to be sent to the two 6-pulse half bridges connected respectively to the Wye(Y) and Delta (D) connected windings of the YYD converter transformer. Pulses are individually synchronized on the 6 commutation voltages and generated alpha degrees after the increasing zero-crossings of the commutation voltages. The D pulses are lagging the Y pulses by  60 degrees.
      |
      | Input 1 is  the alpha firing signal (degrees).
      | Inputs 2, 3 and 4 are the three phase-ground synchronization voltages  measured at the  primary side of the converter transformer.
      | Input 5: Frequency of the synchronization voltages (use a constant or the Freq PLL output)
      | Input 6 allows  blocking of the pulses when the applied signal is non zero.
      |
      | When the 'Douple pulsing' option is checked, two pulses are sent to each thyristor: a 1st pulse when the aplha angle is reached, then a 2nd pulse 60 degrees later, when the next thyristor is fired.
      mask Display: plot(0,0,100,100,[80 62 62 47 47 30],[40 40 60 60 40 40]-5)
  PLL : Subsystem
  PulsesY : Outport
  PulsesD : Outport  Port=2
  Freq : Outport  Port=3
  wires:
  Discrete Synchronized 12-Pulse Generator/1(PY) -> PulsesY/1
  Discrete Synchronized 12-Pulse Generator/2(PD) -> PulsesD/1
  Vabc (pu)/1 -> PLL/1(Vabc(pu))
  PLL/1(Va) -> Discrete Synchronized 12-Pulse Generator/2(A)
  PLL/2(Vb) -> Discrete Synchronized 12-Pulse Generator/3(B)
  PLL/3(Vc) -> Discrete Synchronized 12-Pulse Generator/4(C)
  PLL/4(Freq) -> Discrete Synchronized 12-Pulse Generator/5(Freq), Freq/1
  alpha_ord (deg)/1 -> Discrete Synchronized 12-Pulse Generator/1(alpha_deg)
  Block/1 -> Discrete Synchronized 12-Pulse Generator/6(Block)

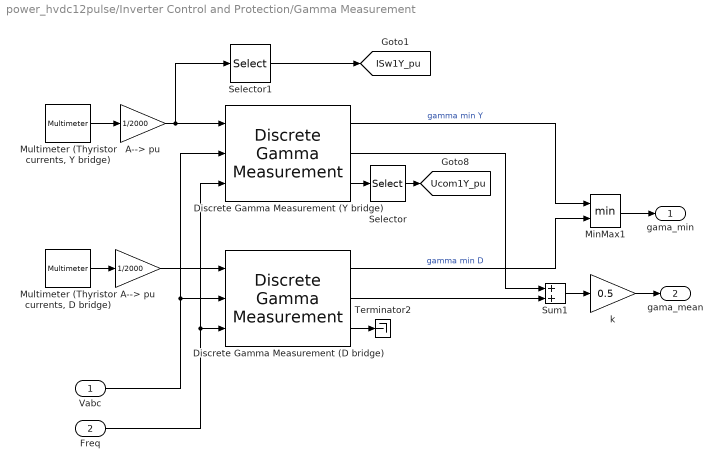
== system power_hvdc12pulse/Inverter Control and Protection/Gamma Measurement ==
  Vabc : Inport  Port=1  LatchInput=off
  Freq : Inport  Port=2  LatchInput=off
  A--> pu : Gain  Gain=1/2000  SaturateOnIntegerOverflow=on
  "A--> pu " : Gain  Gain=1/2000  SaturateOnIntegerOverflow=on
  Discrete Gamma Measurement (D bridge) : powerlib_extras/Discrete  Control Blocks/Discrete Gamma Measurement  transfo_type=Yg / D1(lag)  f0=50  Ith_min=0.001  Ts=Ts
  Discrete Gamma Measurement (Y bridge) : powerlib_extras/Discrete  Control Blocks/Discrete Gamma Measurement  transfo_type=Yg / Y  f0=50  Ith_min=0.001  Ts=Ts
  MinMax1 : MinMax  Inputs=2  SaturateOnIntegerOverflow=on  InputSameDT=on
  "Multimeter (Thyristor currents, D bridge)  " : powerlib/Measurements/Multimeter  Tag=PoWeRsYsTeMmEaSuReMeNt  PhasorSimulation=off  OutputType=Magnitude  sel=[25 26 27 28 29 30]  L=42  Gain=[1 1 1 1 1 1]  yselected={'Isw1: Inverter/Inverter/Bridge D','Isw2: Inverter/Inverter/Bridge D','Isw3: Inverter/Inverter/Bridge D','Isw4: Inverter/Inverter/Bridge D','Isw5: Inverter/Inverter/Bridge D','Isw6: Inverter/Inverter/Bridge D'};  PSBOutputType=1  PSBequivalent=0  AxesSetting=[0,0.1,-100,100]  Display=0  SavedBlockNames=-11
      settings: AttributesFormatString=\n
  "Multimeter (Thyristor currents, Y bridge) " : powerlib/Measurements/Multimeter  Tag=PoWeRsYsTeMmEaSuReMeNt  PhasorSimulation=off  OutputType=Magnitude  sel=[31 32 33 34 35 36]  L=42  Gain=[1 1 1 1 1 1]  yselected={'Isw1: Inverter/Inverter/Bridge Y','Isw2: Inverter/Inverter/Bridge Y','Isw3: Inverter/Inverter/Bridge Y','Isw4: Inverter/Inverter/Bridge Y','Isw5: Inverter/Inverter/Bridge Y','Isw6: Inverter/Inverter/Bridge Y'};  PSBOutputType=1  PSBequivalent=0  AxesSetting=[0,0.1,-100,100]  Display=0  SavedBlockNames=-11
      settings: AttributesFormatString=\n
  Selector : Selector  InputPortWidth=6
  Selector1 : Selector  InputPortWidth=6
  Sum1 : Sum  SaturateOnIntegerOverflow=on  InputSameDT=on
  Terminator2 : Terminator
  k : Gain  Gain=0.5  SaturateOnIntegerOverflow=on
  gama_min : Outport
  gama_mean : Outport  Port=2
  tag scope: ISw1Y_pu=global, Ucom1Y_pu=global
  wires:
  "Multimeter (Thyristor currents, Y bridge) "/1 -> A--> pu/1
  A--> pu/1 -> Selector1/1, Discrete Gamma Measurement (Y bridge)/1
  Vabc/1 -> Discrete Gamma Measurement (Y bridge)/2, Discrete Gamma Measurement (D bridge)/2
  Discrete Gamma Measurement (Y bridge)/1 -> MinMax1/1  "gamma min Y"
  Discrete Gamma Measurement (Y bridge)/3 -> Selector/1
  Discrete Gamma Measurement (Y bridge)/2 -> Sum1/1
  "Multimeter (Thyristor currents, D bridge)  "/1 -> "A--> pu "/1
  "A--> pu "/1 -> Discrete Gamma Measurement (D bridge)/1
  Discrete Gamma Measurement (D bridge)/3 -> Terminator2/1
  Discrete Gamma Measurement (D bridge)/2 -> Sum1/2
  Discrete Gamma Measurement (D bridge)/1 -> MinMax1/2  "gamma min D"
  MinMax1/1 -> gama_min/1
  Sum1/1 -> k/1
  k/1 -> gama_mean/1
  Selector/1 -> [Ucom1Y_pu]
  Selector1/1 -> [ISw1Y_pu]
  Freq/1 -> Discrete Gamma Measurement (Y bridge)/3, Discrete Gamma Measurement (D bridge)/3
